simulink model "HW3_Diff_Eqn"  (R2021b)
settings: Solver=VariableStepAuto  StartTime=0.0  StopTime=10.0  RelTol=1e-3
libraries: simulink x1
settings Model: Creator=rohitkharat  LastModifiedBy=rohitkharat

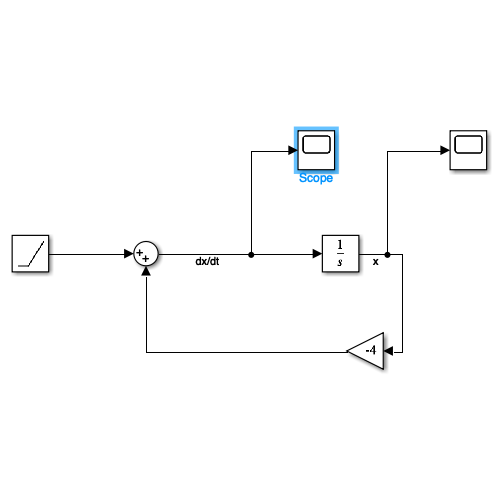
[thumbnail: Simulink's stored preview of the top-level diagram]
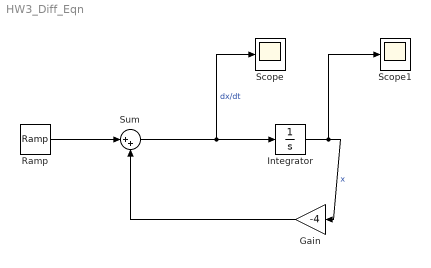
== system HW3_Diff_Eqn ==
  Gain : Gain  Gain=-4
  Integrator : Integrator
  Ramp : simulink/Sources/Ramp  slope=1  start=0  InitialOutput=0
  Scope : Scope
  Scope1 : Scope
  Sum : Sum  Inputs=|++
  wires:
  Sum/1 -> Scope/1, Integrator/1  "dx/dt"
  Integrator/1 -> Scope1/1, Gain/1  "x"
  Gain/1 -> Sum/2
  Ramp/1 -> Sum/1
